simulink model "master"  (R2017a)
settings: Solver=VariableStepAuto  StartTime=0.0  StopTime=10.0  RelTol=1e-3
settings Model: Creator=mini  LastModifiedBy=mini

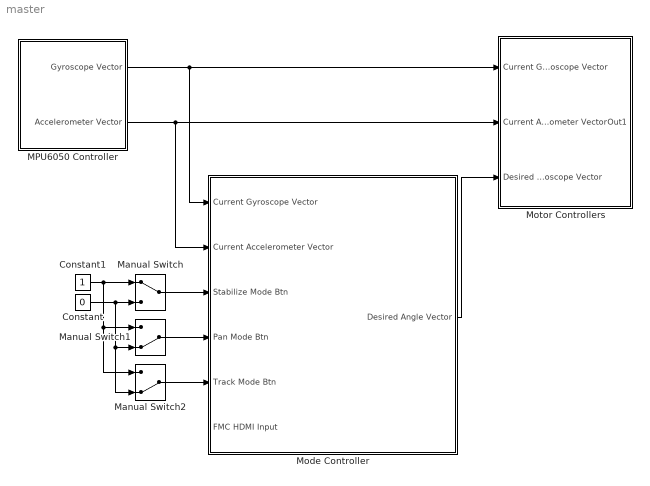
== system master ==
  Constant : Constant  Value=0
  Constant1 : Constant
  MPU6050 Controller : Subsystem
  Manual Switch : ManualSwitch
  Manual Switch1 : ManualSwitch  CurrentSetting=0
  Manual Switch2 : ManualSwitch  CurrentSetting=0
  Mode Controller : Subsystem
  Motor Controllers : Subsystem
  wires:
  MPU6050 Controller/2(Accelerometer Vector) -> Mode Controller/2(Current Accelerometer Vector), Motor Controllers/2(Current Accelerometer Vector)
  MPU6050 Controller/1(Gyroscope Vector) -> Mode Controller/1(Current Gyroscope Vector), Motor Controllers/1(Current Gyroscope Vector)
  Mode Controller/1(Desired Angle Vector) -> Motor Controllers/3(Desired Gyroscope Vector)
  Manual Switch1/1 -> Mode Controller/4(Pan Mode Btn)
  Manual Switch/1 -> Mode Controller/3(Stabilize Mode Btn)
  Manual Switch2/1 -> Mode Controller/5("Track Mode Btn ")
  Constant1/1 -> Manual Switch/1, Manual Switch1/1, Manual Switch2/1
  Constant/1 -> Manual Switch2/2, Manual Switch1/2, Manual Switch/2

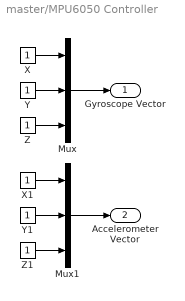
== system master/MPU6050 Controller ==
  Mux : Mux  Inputs=3
  Mux1 : Mux  Inputs=3
  X : Constant
  X1 : Constant
  Y : Constant
  Y1 : Constant
  Z : Constant
  Z1 : Constant
  Gyroscope Vector : Outport
  Accelerometer Vector : Outport  Port=2
  wires:
  X/1 -> Mux/1
  Y/1 -> Mux/2
  Z/1 -> Mux/3
  Mux/1 -> Gyroscope Vector/1
  Y1/1 -> Mux1/2
  Z1/1 -> Mux1/3
  X1/1 -> Mux1/1
  Mux1/1 -> Accelerometer Vector/1

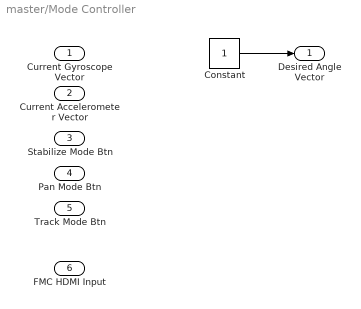
== system master/Mode Controller ==
  Current Gyroscope Vector : Inport
  Current Accelerometer Vector : Inport  Port=2
  Stabilize Mode Btn : Inport  Port=3
  Pan Mode Btn : Inport  Port=4
  "Track Mode Btn " : Inport  Port=5
  FMC HDMI Input : Inport  Port=6
  Constant : Constant
  Desired Angle Vector : Outport
  wires:
  Constant/1 -> Desired Angle Vector/1

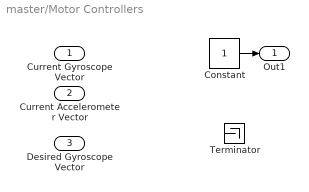
== system master/Motor Controllers ==
  Current Gyroscope Vector : Inport
  Current Accelerometer Vector : Inport  Port=2
  Desired Gyroscope Vector : Inport  Port=3
  Constant : Constant
  Terminator : Terminator
  Out1 : Outport
  wires:
  Constant/1 -> Out1/1
